simulink model "untitled3"  (Simulink 8.8)
settings: Solver=VariableStepAuto  StartTime=0.0  StopTime=20  RelTol=1e-3
libraries: simulink x2
settings Model: Creator=a  LastModifiedBy=a
settings DataIOCC: LimitDataPoints=off  SaveFormat=Dataset  SignalLoggingSaveFormat=Dataset
settings OptimizationCC: LifeSpan=auto
settings DebuggingCC: UnderspecifiedInitializationDetection=Simplified  MergeDetectMultiDrivingBlocksExec=error  FcnCallInpInsideContextMsg=error  StateNameClashWarn=none  SFUnexpectedBacktrackingDiag=error  SFNoUnconditionalDefaultTransitionDiag=error  SFExecutionAtInitializationDiag=warning
settings HardwareCC: ProdBitPerPointer=64  ProdBitPerSizeT=64  ProdBitPerPtrDiffT=64  ProdLargestAtomicFloat=Float  ProdIntDivRoundTo=Zero  ProdEndianess=LittleEndian  ProdWordSize=64  ProdHWDeviceType=Intel->x86-64 (Windows64)
settings ModelReferenceCC: PropagateSignalLabelsOutOfModel=on
settings GRTTargetCC: TargetLangStandard=C99 (ISO)  GeneratePreprocessorConditionals=Use local settings  CombineOutputUpdateFcns=on  GRTInterface=off
settings ConfigComp: CovMetricSettings=dwe  CovHtmlReporting=off  CovSaveCumulativeToWorkspaceVar=off  CovSaveSingleToWorkspaceVar=off  CovExternalEMLEnable=on

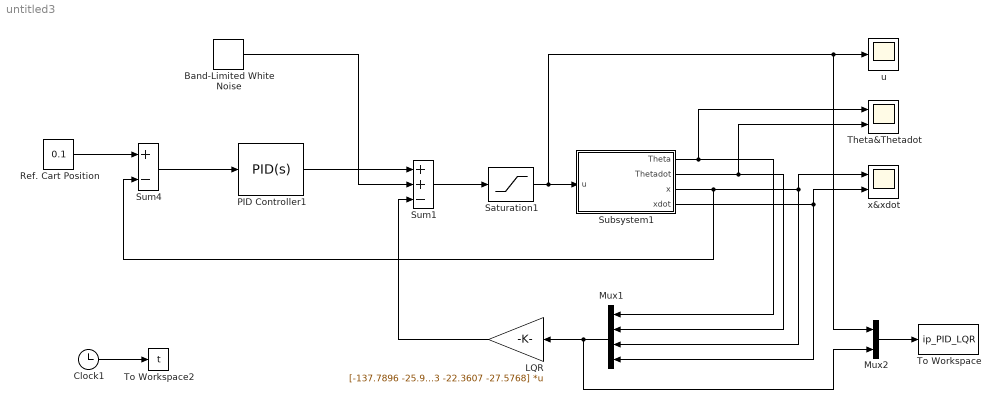
== system untitled3 ==
  Band-Limited White Noise : simulink/Sources/Band-Limited White Noise  Cov=[0.001]  Ts=0.01  seed=[23341]
  Clock1 : Clock
  LQR : Gain  Gain=[-137.7896 -25.9783 -22.3607 -27.5768]  Multiplication=Matrix(K*u)
  Mux1 : Mux
  Mux2 : Mux  Inputs=2
  PID Controller1 : simulink/Continuous/PID Controller  Controller=PID  TimeDomain=Continuous-time  SampleTime=-1  IntegratorMethod=Forward Euler  FilterMethod=Forward Euler  Form=Parallel  UseFilter=on  ControllerParametersSource=internal  P=1.5  I=-7.5  D=5  N=100  InitialConditionSource=internal  InitialConditionForIntegrator=0  InitialConditionForFilter=0  ExternalReset=none  LimitOutput=off  UpperSaturationLimit=inf  LowerSaturationLimit=-inf  LinearizeAsGain=off  AntiWindupMode=none  Kb=1  TrackingMode=off  Kt=1  PParamMin=[]  PParamMax=[]  IParamMin=[]  IParamMax=[]  DParamMin=[]  DParamMax=[]  NParamMin=[]  NParamMax=[]  KbParamMin=[]  KbParamMax=[]  KtParamMin=[]  KtParamMax=[]  POutMin=[]  POutMax=[]  IOutMin=[]  IOutMax=[]  DOutMin=[]  DOutMax=[]  NOutMin=[]  NOutMax=[]  KbOutMin=[]  KbOutMax=[]  KtOutMin=[]  KtOutMax=[]  IntegratorOutMin=[]  IntegratorOutMax=[]  FilterOutMin=[]  FilterOutMax=[]  SumOutMin=[]  SumOutMax=[]  SumI1OutMin=[]  SumI1OutMax=[]  SumI2OutMin=[]  SumI2OutMax=[]  SumI3OutMin=[]  SumI3OutMax=[]  SumDOutMin=[]  SumDOutMax=[]  SaturationOutMin=[]  SaturationOutMax=[]  IntegratorContinuousStateAttributes=''  IntegratorStateMustResolveToSignalObject=off  IntegratorRTWStateStorageClass=Auto  FilterContinuousStateAttributes=''  FilterStateMustResolveToSignalObject=off  FilterRTWStateStorageClass=Auto  DifferentiatorICPrevScaledInput=0  DifferentiatorOutMin=[]  DifferentiatorOutMax=[]
  Ref. Cart Position : Constant  Value=0.1
  Saturation1 : Saturate  UpperLimit=100  LowerLimit=-100
  Subsystem1 : Subsystem
  Sum1 : Sum  Inputs=++-  SaturateOnIntegerOverflow=on  InputSameDT=on  OutDataTypeStr=Inherit: Same as first input
  Sum4 : Sum  Inputs=+-  SaturateOnIntegerOverflow=on  InputSameDT=on  OutDataTypeStr=Inherit: Same as first input
  Theta&Thetadot : Scope  NumInputPorts=2
  To Workspace : ToWorkspace  VariableName=ip_PID_LQR  SampleTime=-1
  To Workspace2 : ToWorkspace  VariableName=t  SampleTime=-1
  u : Scope
  x&xdot : Scope  NumInputPorts=2
  wires:
  Subsystem1/2(Thetadot) -> Mux1/2, Theta&Thetadot/2
  Subsystem1/3(x) -> Mux1/3, x&xdot/1, Sum4/2
  Subsystem1/4(xdot) -> Mux1/4, x&xdot/2
  Mux1/1 -> LQR/1, Mux2/2
  Sum1/1 -> Saturation1/1
  Saturation1/1 -> u/1, Mux2/1, Subsystem1/1(u)
  Sum4/1 -> PID Controller1/1
  Ref. Cart Position/1 -> Sum4/1
  Clock1/1 -> To Workspace2/1
  Mux2/1 -> To Workspace/1
  PID Controller1/1 -> Sum1/1
  Subsystem1/1(Theta) -> Mux1/1, Theta&Thetadot/1
  LQR/1 -> Sum1/3
  Band-Limited White Noise/1 -> Sum1/2

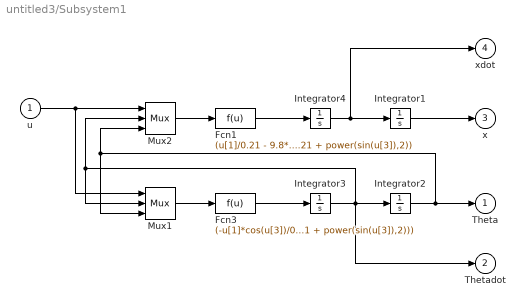
== system untitled3/Subsystem1 ==
  u : Inport
  Fcn1 : Fcn  Expr=(u[1]/0.21 - 9.8*sin(u[3])*cos(u[3]) + (0.61/2)*power(u[2],2)*sin(u[3]))/(0.455/0.21 + power(sin(u[3]),2))
  Fcn3 : Fcn  Expr=(-u[1]*cos(u[3])/0.21 + (0.455+0.21)*9.8*sin(u[3])/0.21 - (0.61/2)*power(u[2],2)*sin(u[3])*cos(u[3]))/((0.61/2)*(0.455/0.21 + power(sin(u[3]),2)))
  Integrator{1..4} (4 alike) : Integrator
  Mux1 : Mux  Inputs=3
  Mux2 : Mux  Inputs=3
  Theta : Outport  InitialOutput=0
  Thetadot : Outport  Port=2  InitialOutput=0
  x : Outport  Port=3  InitialOutput=0
  xdot : Outport  Port=4  InitialOutput=0
  wires:
  Integrator1/1 -> x/1
  Fcn3/1 -> Integrator3/1
  Mux1/1 -> Fcn3/1
  Mux2/1 -> Fcn1/1
  Fcn1/1 -> Integrator4/1
  Integrator4/1 -> Integrator1/1, xdot/1
  u/1 -> Mux2/1, Mux1/1
  Integrator3/1 -> Integrator2/1, Mux2/2, Mux1/2, Thetadot/1
  Integrator2/1 -> Theta/1, Mux2/3, Mux1/3
